simulink model "LQR_bloques_SS_gamma"  (R2023a)
settings: Solver=VariableStepAuto  StartTime=0.0  StopTime=500  RelTol=1e-6
undefined symbols (not defined in the file): A, A_model, A_motor, B, B_mag0, B_model, B_model2, B_motor, C_model, C_model2, C_motor, D_model, D_motor, Gamma, I, J, juliandate, K1, K1_2, K2, K2_2, K3, K_gamma, Ke, Kt, La, n_cal, R_mgt, Ra, T_ext, T_max, T_max_mgt, x0
libraries: slpidlib x12, matrix_library x10, simulink_extras x5, sharedutil x3, aerolibutil x2, vrlib x2, aerolibcubesatveh x1, aerolibgravity2 x1
(part 1 of 2)
settings Model: Creator=Personal  LastModifiedBy=ASUS
settings SolverCC: ZeroCrossAlgorithm=Adaptive
settings DebuggingCC: MaskedZcDiagnostic=none  IgnoredZcDiagnostic=none

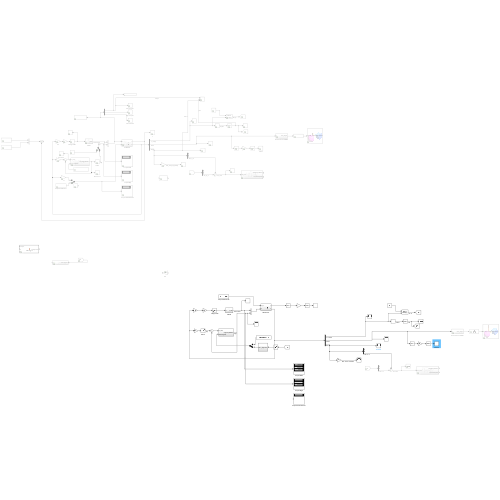
[thumbnail: Simulink's stored preview of the top-level diagram]
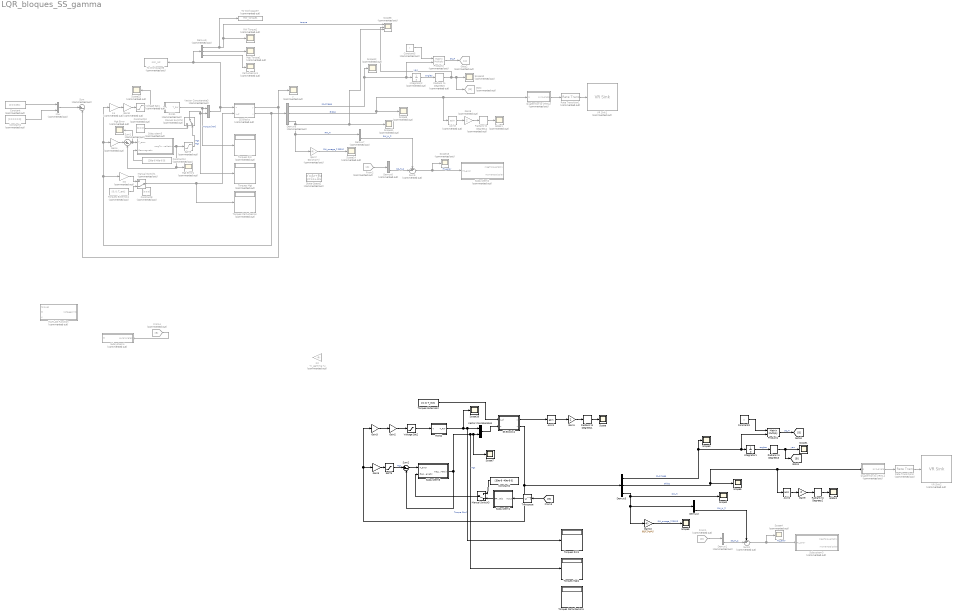
== system LQR_bloques_SS_gamma ==
  Asin1 : Trigonometry  Operator=asin
  Asin2 : Trigonometry  Operator=asin
  Asin3 : Trigonometry  Commented=on  Operator=asin
  Constant : Constant  Commented=on  Value=[0 0 0.05 ]
  Constant1 : Constant  Commented=on  Value=[0 0 0 0 0 0]
  Constant10 : Constant  Commented=on  Value=[0;0;0]
  Constant12 : Constant  Commented=on  Value=[30e-6 40e-6 0]
  Constant2 : Constant  Value=[30e-6 -40e-6 0]
  Constant3 : Constant  Value=I
  Constant5 : Constant  Commented=on  Value=I
  Constant8 : Constant  Commented=on  Value=[0;0;0]
  Demux{1,6..9} (5 alike) : Demux  Commented=on  Outputs=3
  Demux2 : Demux  Outputs=3
  Demux3 : Demux  Outputs=3
  From1 : From  Commented=on  GotoTag=D
  From2 : From  Commented=on
  From4 : From  Commented=on  GotoTag=B
  Gain1 : Gain  Gain=2
  Gain10 : Gain  Gain=60/(2*pi*J)
  Gain2 : Gain  Gain=Ra/Kt
  Gain3 : Gain  Gain=-K1_2  Multiplication=Matrix(K*u)
  Gain4 : Gain  Commented=on  Gain=-K2  Multiplication=Matrix(K*u)
  Gain5 : Gain  Gain=-K2_2  Multiplication=Matrix(K*u)
  Gain6 : Gain  Commented=on  Gain=2
  Gain7 : Gain  Commented=on  Gain=60/(2*pi*J)
  Gain8 : Gain  Commented=on  Gain=Ra/Kt
  Gain9 : Gain  Gain=2
  Gibbs1 : Scope  Commented=on
  Gibbs2 : Scope
  Goto : Goto  Commented=on  GotoTag=B
  Goto2 : Goto  Commented=on
  Integrator1 : Integrator  InitialCondition=[0 0 0]
  Integrator2 : Integrator  Commented=on  InitialCondition=[0 0 0]
  K2 : Gain  Commented=on  Gain=-K_gamma  Multiplication=Matrix(K*u)
  K4 : Gain  Commented=on  Gain=-K1  Multiplication=Matrix(K*u)
  K6 : Gain  Commented=on  Gain=-K3  Multiplication=Matrix(K*u)
  MATLAB Function : MATLAB Function  Commented=on  TreatAsAtomicUnit=on
  Manual Switch1 : ManualSwitch  Commented=on  CurrentSetting=0
  Manual Switch2 : ManualSwitch  Commented=on  CurrentSetting=0
  Manual Switch3 : ManualSwitch  CurrentSetting=0
  Mgt Error : Scope  Commented=on
  Mgt Error1 : Scope  Commented=on
  Mgt Torque1 : Scope  Commented=on
  Mux : Mux  Commented=on  Inputs=2
  Perturbacion1 : Scope  Commented=on
  Product1 : Product  Multiplication=Matrix(*)
  Product2 : Product  Commented=on  Multiplication=Matrix(*)
  Quaternion to VRML1 : Subsystem  Commented=on
  Quaternion to VRML2 : Subsystem  Commented=on
  RW Torque1 : Scope  Commented=on
  RWS1 : Subsystem  Commented=on
  RWS2 : Subsystem
  Radians to Degrees1 : simulink_extras/Transformations/Radians to Degrees
  Radians to Degrees2 : simulink_extras/Transformations/Radians to Degrees
  Radians to Degrees3 : simulink_extras/Transformations/Radians to Degrees
  Radians to Degrees4 : simulink_extras/Transformations/Radians to Degrees  Commented=on
  Radians to Degrees5 : simulink_extras/Transformations/Radians to Degrees  Commented=on
  Rate Transition1 : RateTransition  Commented=on
  Rate Transition2 : RateTransition  Commented=on
  SS Blocks : Subsystem  Commented=on
  SS Blocks1 : Subsystem
  SatT3 : Saturate  Commented=on  UpperLimit=T_max_mgt  LowerLimit=-T_max_mgt
  SatT5 : Saturate  UpperLimit=T_max_mgt  LowerLimit=-T_max_mgt
  Scope{,1..3,5..7,16} (8 alike) : Scope
  Scope{4,9..15} (8 alike) : Scope  Commented=on
  Scope8 : Scope  Commented=on  NumInputPorts=3
  State-Space2 : StateSpace  Commented=on  A=A_model  B=B_model  C=C_model  D=D_model  InitialCondition=x0
  Subsystem1 : Subsystem
  Subsystem2 : Subsystem  Commented=on
  Subsystem3 : Subsystem  Commented=on
  Subsystem4 : Subsystem  Commented=on
  Subsystem5 : Subsystem  Commented=on
  Subsystem6 : Subsystem
  Sum : Sum  Commented=on  Inputs=|+-
  Sum1 : Sum  Commented=on  Inputs=|+-
  Sum2 : Sum  Inputs=|+-
  Sum3 : Sum  Commented=on  Inputs=+-|
  Sum5 : Sum  Commented=on  Inputs=+-|
  To Workspace6 : ToWorkspace  Commented=on  VariableName=sim_U2  SaveFormat=Structure With Time  SampleTime=-1
  To Workspace7 : ToWorkspace  Commented=on  VariableName=RW_torque1  SaveFormat=Structure With Time  SampleTime=-1
  Torques Externos1 : Constant  Commented=on  Value=[0; 0; T_ext]
  Torques Externos2 : Constant  Value=[0; 0; T_ext]
  Torques Mgt : Display  Commented=on
  Torques Mgt1 : Display
  Torques Perturbacion : Display  Commented=on
  Torques Perturbacion1 : Display
  Torques RW : Display  Commented=on
  Torques RW1 : Display
  Transpose : Math  Operator=transpose
  VR Sink1 : vrlib/VR Sink  Commented=on  InstantiateOnLoad=on  SampleTime=0.1  ViewEnable=on  RemoteChange=off  RemoteView=off  FieldsWritten=STLB_Transform.rotation.4.1.1.double  WorldFileName=EscenarioCubeSat.x3d  AutoView=off  VideoDimensions=[]  AllowVariableSize=off  FigureProperties=[]
  VR Sink2 : vrlib/VR Sink  Commented=on  InstantiateOnLoad=on  SampleTime=0.1  ViewEnable=on  RemoteChange=off  RemoteView=off  FieldsWritten=STLB_Transform.rotation.4.1.1.double  WorldFileName=EscenarioCubeSat.x3d  AutoView=off  VideoDimensions=[]  AllowVariableSize=off  FigureProperties=[]
  Vector Concatenate1 : Concatenate
  Vector Concatenate3 : Concatenate  Commented=on
  Voltage Sat1 : Saturate  Commented=on  UpperLimit=6  LowerLimit=-6
  Voltage Sat2 : Saturate  UpperLimit=6  LowerLimit=-6
  y : Scope  Commented=on
  wires:
  Integrator2/1 -> Radians to Degrees5/1  "angles"
  Gain7/1 -> Scope14/1  "RW_omega_Z [RPM]"
  Constant5/1 -> Product2/1
  From4/1 -> Subsystem4/1(euler angles)
  SatT3/1 -> Manual Switch2/2  "Mgt"
  Gain8/1 -> Voltage Sat1/1
  Quaternion to VRML2/1(axis_angle) -> Rate Transition1/1
  From2/1 -> Demux6/1
  Constant10/1 -> Manual Switch2/1
  Asin3/1 -> Gain6/1
  Product2/1 -> Goto2/1  "SC_H"
  Radians to Degrees5/1 -> Scope8/2, Goto/1, Scope10/1  "yaw"
  Demux8/3 -> Scope8/3, Scope11/1, Gain7/1, Demux7/1  "RW_H"
  Demux8/1 -> Integrator2/1, Product2/2, Scope12/1  "sc_omega"
  Voltage Sat1/1 -> Scope15/1, RWS1/1(V)
  Demux7/3 -> Sum5/1  "RW_H_Z"
  Radians to Degrees4/1 -> Gibbs1/1
  Demux9/1 -> To Workspace7/1, Scope8/1, RW Torque1/1  "torque"
  K4/1 -> Gain8/1
  Torques Externos1/1 -> Manual Switch1/2
  Sum5/1 -> Scope13/1, Subsystem2/1(Hz_error)  "Hz_error"
  Demux6/3 -> Sum5/2  "SC_H_Z"
  Rate Transition1/1 -> VR Sink1/1
  Gain6/1 -> Radians to Degrees4/1
  Demux8/2 -> Asin3/1, Quaternion to VRML2/1(q), Scope9/1  "Gibbs"
  RWS1/1(T_RW) -> Torques RW/1, Vector Concatenate3/1  "Torque [Nm]"
  Demux9/2 -> Mgt Torque1/1
  K6/1 -> Manual Switch1/1
  Demux9/3 -> Perturbacion1/1
  Vector Concatenate3/1 -> To Workspace6/1, Demux9/1, SS Blocks/1(u)
  Manual Switch2/1 -> Vector Concatenate3/2, Torques Mgt/1  "Mgt"
  Manual Switch1/1 -> SS Blocks/2(u_d), Torques Perturbacion/1
  SS Blocks/2(x) -> K6/1, K4/1, Gain4/1, Demux8/1
  SS Blocks/1(y) -> Sum/2, y/1
  Constant/1 -> Mux/1
  Constant1/1 -> Mux/2
  Mux/1 -> Sum/1
  Sum1/1 -> Mgt Error/1, Subsystem5/1(T_error)
  Gain4/1 -> Sum1/1
  Subsystem5/1(magTorqueMatrix) -> SatT3/1, Mgt Error1/1, Sum1/2
  Constant12/1 -> Subsystem5/2(Geomagnetic)
  Torques Externos2/1 -> SS Blocks1/1(u_d)
  SS Blocks1/1(y) -> Asin1/1
  Gain1/1 -> Radians to Degrees1/1
  Asin1/1 -> Gain1/1
  Radians to Degrees1/1 -> Scope/1
  SS Blocks1/2(x) -> Demux3/1, Gain3/1, Gain5/1
  Gain5/1 -> SatT5/1
  Gain3/1 -> Gain2/1
  Gain2/1 -> Voltage Sat2/1
  Voltage Sat2/1 -> RWS2/1(V)
  RWS2/1(T_RW) -> Scope16/1, Torques RW1/1, Vector Concatenate1/1  "Torque [Nm]"
  Sum2/1 -> Subsystem6/1(T_error)
  Subsystem6/1(magTorqueMatrix) -> Sum2/2, Torques Mgt1/1, Scope7/1, Vector Concatenate1/2  "Mgt"
  Vector Concatenate1/1 -> SS Blocks1/2(u)
  Demux2/3 -> Sum3/1  "RW_H_Z"
  Demux3/1 -> Integrator1/1, Product1/2, Scope3/1  "sc_omega"
  Demux3/3 -> Scope2/1, Gain10/1, Demux2/1  "RW_H"
  Sum3/1 -> Scope4/1, Subsystem3/1(Hz_error)  "Hz_error"
  Gain9/1 -> Radians to Degrees2/1
  Demux1/3 -> Sum3/2  "SC_H_Z"
  Product1/1 -> [D]  "SC_H"
  Demux3/2 -> Asin2/1, Quaternion to VRML1/1(q), Scope6/1  "Gibbs"
  Radians to Degrees2/1 -> Gibbs2/1
  Rate Transition2/1 -> VR Sink2/1
  Quaternion to VRML1/1(axis_angle) -> Rate Transition2/1
  Constant3/1 -> Product1/1
  Asin2/1 -> Gain9/1
  Radians to Degrees3/1 -> [B], Scope1/1  "yaw"
  From1/1 -> Demux1/1
  Gain10/1 -> Scope5/1  "RW_omega_Z [RPM]"
  Integrator1/1 -> Radians to Degrees3/1  "angles"
  SatT5/1 -> Sum2/1  "Mgt"
  Constant2/1 -> Manual Switch3/1
  Manual Switch3/1 -> Subsystem6/2(Geomagnetic)
  Subsystem1/1(RPY_Magnetic) -> Manual Switch3/2
  Transpose/1 -> Subsystem1/1(Input)
  [B] -> Transpose/1

== system LQR_bloques_SS_gamma/Quaternion to VRML1 ==
  q : Inport
  Asin1 : Trigonometry  Operator=asin
  Constant : Constant  Value=pi/2
  Demux : Demux  Outputs=3
  "Flip 180 deg, rotate 90" : Constant  Value=[0 0.2 0 0]
  Gain2 : Gain  Gain=2
  Mux : Mux
  Quaternion Multiplication : aerolibutil/Quaternion Multiplication
  Saturation : Saturate
  Selector1 : Selector  InputPortWidth=4  IndexOptions=Index vector (dialog)  Indices=[2 3 1 4]  OutputSizes=1
  Sum : Sum  Inputs=|+-
  axis_angle : Outport  VectorParamsAs1DForOutWhenUnconnected=off
  wires:
  Constant/1 -> Sum/1
  Saturation/1 -> Asin1/1
  Asin1/1 -> Gain2/1
  Demux/3 -> Mux/3, Saturation/1
  Gain2/1 -> Mux/4
  Selector1/1 -> axis_angle/1
  Mux/1 -> Selector1/1
  Demux/1 -> Mux/1
  q/1 -> Demux/1
  "Flip 180 deg, rotate 90"/1 -> Quaternion Multiplication/2
  Demux/2 -> Mux/2

== system LQR_bloques_SS_gamma/Quaternion to VRML2 ==
  q : Inport
  Asin1 : Trigonometry  Operator=asin
  Constant : Constant  Value=pi/2
  Demux : Demux  Outputs=3
  "Flip 180 deg, rotate 90" : Constant  Value=[0 0.2 0 0]
  Gain2 : Gain  Gain=2
  Mux : Mux
  Quaternion Multiplication : aerolibutil/Quaternion Multiplication
  Saturation : Saturate
  Selector1 : Selector  InputPortWidth=4  IndexOptions=Index vector (dialog)  Indices=[2 3 1 4]  OutputSizes=1
  Sum : Sum  Inputs=|+-
  axis_angle : Outport  VectorParamsAs1DForOutWhenUnconnected=off
  wires:
  Constant/1 -> Sum/1
  Saturation/1 -> Asin1/1
  Asin1/1 -> Gain2/1
  Demux/3 -> Mux/3, Saturation/1
  Gain2/1 -> Mux/4
  Selector1/1 -> axis_angle/1
  Mux/1 -> Selector1/1
  Demux/1 -> Mux/1
  q/1 -> Demux/1
  "Flip 180 deg, rotate 90"/1 -> Quaternion Multiplication/2
  Demux/2 -> Mux/2

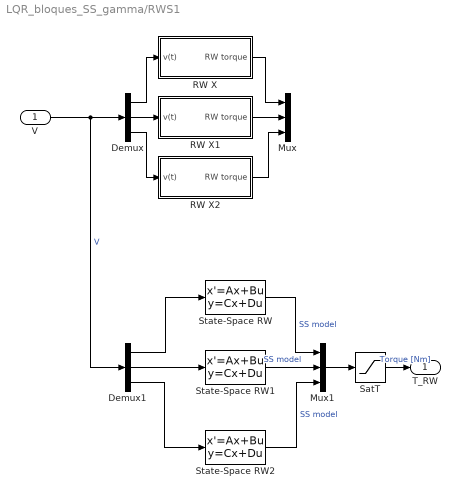
== system LQR_bloques_SS_gamma/RWS1 ==
  V : Inport
  Demux : Demux  Outputs=3
  Demux1 : Demux  Outputs=3
  Mux : Mux  Inputs=3
  Mux1 : Mux  Inputs=3
  RW X : Subsystem
  RW X1 : Subsystem
  RW X2 : Subsystem
  SatT : Saturate  UpperLimit=T_max  LowerLimit=-T_max
  State-Space RW : StateSpace  A=A_motor  B=B_motor  C=C_motor  D=D_motor  InitialCondition=0
  State-Space RW1 : StateSpace  A=A_motor  B=B_motor  C=C_motor  D=D_motor  InitialCondition=0
  State-Space RW2 : StateSpace  A=A_motor  B=B_motor  C=C_motor  D=D_motor  InitialCondition=0
  T_RW : Outport
  wires:
  Demux/1 -> RW X/1(v(t))
  V/1 -> Demux1/1, Demux/1  "V"
  Demux/3 -> RW X2/1(v(t))
  Demux/2 -> RW X1/1(v(t))
  RW X1/1(RW torque) -> Mux/2
  RW X2/1(RW torque) -> Mux/3
  RW X/1(RW torque) -> Mux/1
  Demux1/1 -> State-Space RW/1
  Demux1/2 -> State-Space RW1/1
  Demux1/3 -> State-Space RW2/1
  State-Space RW1/1 -> Mux1/2  "SS model"
  State-Space RW/1 -> Mux1/1  "SS model"
  State-Space RW2/1 -> Mux1/3  "SS model"
  Mux1/1 -> SatT/1
  SatT/1 -> T_RW/1  "Torque [Nm]"

== system LQR_bloques_SS_gamma/RWS2 ==
  V : Inport
  Demux : Demux  Outputs=3
  Demux1 : Demux  Outputs=3
  Mux : Mux  Inputs=3
  Mux1 : Mux  Inputs=3
  RW X : Subsystem
  RW X1 : Subsystem
  RW X2 : Subsystem
  SatT : Saturate  UpperLimit=T_max  LowerLimit=-T_max
  State-Space RW : StateSpace  A=A_motor  B=B_motor  C=C_motor  D=D_motor  InitialCondition=0
  State-Space RW1 : StateSpace  A=A_motor  B=B_motor  C=C_motor  D=D_motor  InitialCondition=0
  State-Space RW2 : StateSpace  A=A_motor  B=B_motor  C=C_motor  D=D_motor  InitialCondition=0
  T_RW : Outport
  wires:
  Demux/1 -> RW X/1(v(t))
  V/1 -> Demux1/1, Demux/1  "V"
  Demux/3 -> RW X2/1(v(t))
  Demux/2 -> RW X1/1(v(t))
  RW X1/1(RW torque) -> Mux/2
  RW X2/1(RW torque) -> Mux/3
  RW X/1(RW torque) -> Mux/1
  Demux1/1 -> State-Space RW/1
  Demux1/2 -> State-Space RW1/1
  Demux1/3 -> State-Space RW2/1
  State-Space RW1/1 -> Mux1/2  "SS model"
  State-Space RW/1 -> Mux1/1  "SS model"
  State-Space RW2/1 -> Mux1/3  "SS model"
  Mux1/1 -> SatT/1
  SatT/1 -> T_RW/1  "Torque [Nm]"

== system LQR_bloques_SS_gamma/SS Blocks ==
  u : Inport
  u_d : Inport  Port=2
  A : Gain  Gain=A_model  Multiplication=Matrix(K*u)
  B : Gain  Gain=B_model2  Multiplication=Matrix(K*u)
  B1 : Gain  Gain=Gamma  Multiplication=Matrix(K*u)
  C : Gain  Gain=C_model2  Multiplication=Matrix(K*u)
  Integrator : Integrator  InitialCondition=x0
  Sum : Sum  Inputs=+++
  y : Outport
  x : Outport  Port=2
  wires:
  B/1 -> Sum/2
  u/1 -> B/1
  Sum/1 -> Integrator/1  "x_dot"
  A/1 -> Sum/3
  C/1 -> y/1
  Integrator/1 -> C/1, x/1, A/1
  u_d/1 -> B1/1
  B1/1 -> Sum/1

== system LQR_bloques_SS_gamma/SS Blocks1 ==
  u_d : Inport
  u : Inport  Port=2
  A : Gain  Gain=A_model  Multiplication=Matrix(K*u)
  B : Gain  Gain=B_model2  Multiplication=Matrix(K*u)
  C : Gain  Gain=C_model2  Multiplication=Matrix(K*u)
  Gamma : Gain  Gain=Gamma  Multiplication=Matrix(K*u)
  Integrator : Integrator  InitialCondition=x0
  Sum : Sum  Inputs=+++
  y : Outport
  x : Outport  Port=2
  wires:
  B/1 -> Sum/2
  u/1 -> B/1
  Sum/1 -> Integrator/1  "x_dot"
  A/1 -> Sum/3
  C/1 -> y/1
  Integrator/1 -> C/1, x/1, A/1
  u_d/1 -> Gamma/1
  Gamma/1 -> Sum/1

== system LQR_bloques_SS_gamma/Subsystem1 ==
  Input : Inport
  Clock : Clock
  Constant1 : Constant  Value=B_mag0
  Extract B : MATLAB Function  TreatAsAtomicUnit=on
  MATLAB Function : MATLAB Function  TreatAsAtomicUnit=on
  Scope8 : Scope
  Zero-Order Hold : ZeroOrderHold  SampleTime=-1
  RPY_Magnetic : Outport
  wires:
  Constant1/1 -> Extract B/1(B_cal)
  Extract B/1(XYZ_Magnetic) -> MATLAB Function/1(NEDMagnetic), Scope8/1
  Input/1 -> MATLAB Function/2(RPY)
  Zero-Order Hold/1 -> Extract B/2(time)
  MATLAB Function/1(RPY_Magnetic) -> RPY_Magnetic/1
  Clock/1 -> Zero-Order Hold/1

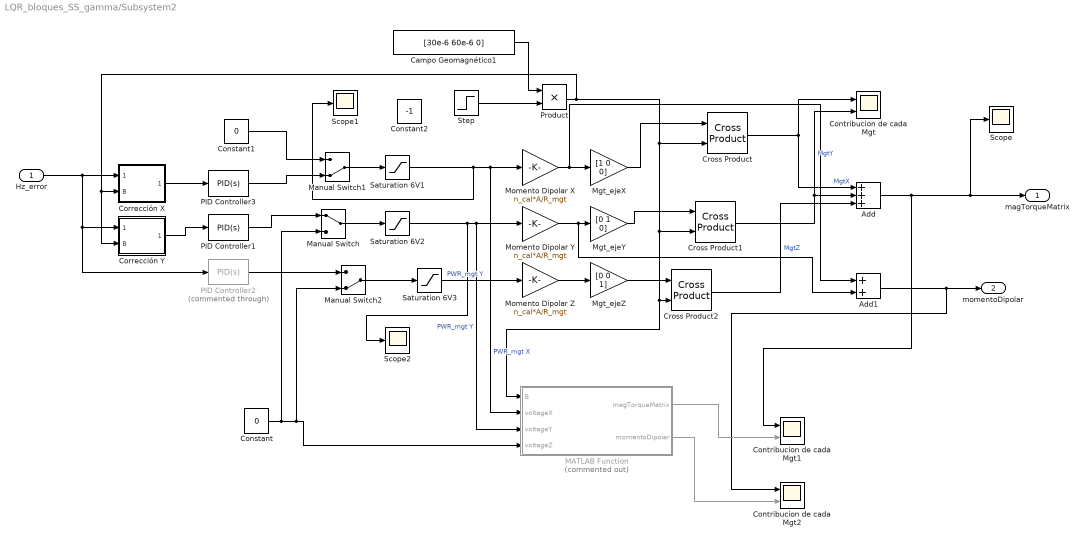
== system LQR_bloques_SS_gamma/Subsystem2 ==
  Hz_error : Inport
  Add : Sum  Inputs=+++
  Add1 : Sum
  Campo Geomagnético1 : Constant  Value=[30e-6 60e-6 0]
  Constant : Constant  Value=0
  Constant1 : Constant  Value=0
  Constant2 : Constant  Value=-1
  Contribucion de cada Mgt : Scope  NumInputPorts=2
  Contribucion de cada Mgt1 : Scope  NumInputPorts=2
  Contribucion de cada Mgt2 : Scope  NumInputPorts=2
  Corrección X : MATLAB Function  TreatAsAtomicUnit=on
  Corrección Y : MATLAB Function  TreatAsAtomicUnit=on
  Cross Product : matrix_library/Cross Product
  Cross Product1 : matrix_library/Cross Product
  Cross Product2 : matrix_library/Cross Product
  MATLAB Function : MATLAB Function  Commented=on  TreatAsAtomicUnit=on
  Manual Switch : ManualSwitch
  Manual Switch1 : ManualSwitch  CurrentSetting=0
  Manual Switch2 : ManualSwitch  CurrentSetting=0
  Mgt_ejeX : Gain  Gain=[1 0 0]
  Mgt_ejeY : Gain  Gain=[0 1 0]
  Mgt_ejeZ : Gain  Gain=[0 0 1]
  Momento Dipolar X : Gain  Gain=n_cal*A/R_mgt
  Momento Dipolar Y : Gain  Gain=n_cal*A/R_mgt
  Momento Dipolar Z : Gain  Gain=n_cal*A/R_mgt
  PID Controller1 : slpidlib/PID Controller  Controller=PID  Form=Parallel  TimeDomain=Continuous-time  UseExternalTs=off  SampleTime=-1  IntegratorMethod=Forward Euler  FilterMethod=Forward Euler  ControllerParametersSource=internal  P=4500  I=800  UseKiTs=off  D=8000  N=100  UseFilter=on  TunerSelectOption=Transfer Function Based (PID Tuner App)  InitialConditionSource=internal  InitialConditionForIntegrator=0  InitialConditionForFilter=0  DifferentiatorICPrevScaledInput=0  ExternalReset=none  TrackingMode=off  Kt=1  LimitOutput=off  SatLimitsSource=internal  UpperSaturationLimit=1  LowerSaturationLimit=-1  LinearizeAsGain=on  AntiWindupMode=none  Kb=1  LimitIntegrator=off  UpperIntegratorSaturationLimit=inf  LowerIntegratorSaturationLimit=-inf  POutMin=[]  POutMax=[]  IOutMin=[]  IOutMax=[]  DOutMin=[]  DOutMax=[]  NOutMin=[]  NOutMax=[]  SumOutMin=[]  SumOutMax=[]  SaturationOutMin=[]  SaturationOutMax=[]  PParamMin=[]  PParamMax=[]  IParamMin=[]  IParamMax=[]  DParamMin=[]  DParamMax=[]  NParamMin=[]  NParamMax=[]  KbParamMin=[]  KbParamMax=[]  KtParamMin=[]  KtParamMax=[]  KbOutMin=[]  KbOutMax=[]  KtOutMin=[]  KtOutMax=[]  IntegratorOutMin=[]  IntegratorOutMax=[]  FilterOutMin=[]  FilterOutMax=[]  SumI1OutMin=[]  SumI1OutMax=[]  SumI2OutMin=[]  SumI2OutMax=[]  SumI3OutMin=[]  SumI3OutMax=[]  SumI4OutMin=[]  SumI4OutMax=[]  SumDOutMin=[]  SumDOutMax=[]  DifferentiatorOutMin=[]  DifferentiatorOutMax=[]  FilterDiffOutCoefMin=[]  FilterDiffOutCoefMax=[]  ReciprocalOutMin=[]  ReciprocalOutMax=[]  SumDenOutMin=[]  SumDenOutMax=[]  SumNumOutMin=[]  SumNumOutMax=[]  DivideOutMin=[]  DivideOutMax=[]  UdiffTsProdOutMin=[]  UdiffTsProdOutMax=[]  NTsProdOutMin=[]  NTsProdOutMax=[]  UintegralTsProdOutMin=[]  UintegralTsProdOutMax=[]  UngainTsProdOutMin=[]  UngainTsProdOutMax=[]  ClampingZeroOutDataTypeStr=Inherit: Inherit via back propagation  ClampingZeroOutMin=[]  ClampingZeroOutMax=[]  FilterDenConstantOutDataTypeStr=Inherit: Inherit via back propagation  FilterDenConstantOutMin=[]  FilterDenConstantOutMax=[]  PCopyOutDataTypeStr=Inherit: Inherit via back propagation  PCopyOutMin=[]  PCopyOutMax=[]  NCopyOutDataTypeStr=Inherit: Inherit via back propagation  NCopyOutMin=[]  NCopyOutMax=[]  IntegratorContinuousStateAttributes=''  IntegratorStateMustResolveToSignalObject=off  IntegratorRTWStateStorageClass=Auto  FilterContinuousStateAttributes=''  FilterStateMustResolveToSignalObject=off  FilterRTWStateStorageClass=Auto  ParallelPVariant=InternalParameters  IdealPVariant=Disabled  IVariant=InternalParameters  DVariant=InternalParameters  IntegratorVariant=Continuous  SatVariant=Disabled  AWVariant=Passthrough  PCopyVariant=Disabled  TRVariant=Disabled  FdbkBlocksVariant=Forward  IdealPFdbkVariant=Disabled  SatFdbkVariant=Disabled  DerivativeFilterVariant=ContFilter  NVariant=InternalParameters  NCopyVariant=Disabled  FilterICVariant=InternalICsFilter  IntegratorICVariant=InternalICs  ExternalResetVariant=Disabled  TRSumVariant=Passthrough  SumFdbkVariant=Disabled  SumVariant=Sum_PID  TsampFilterVariant=InternalTs  TsampNgainVariant=Passthrough  TsampIntegralVariant=Disabled_SignalSpec  ExternalSaturationOutDataTypeStr=Inherit: Same as second input
  PID Controller2 : slpidlib/PID Controller  Commented=through  Controller=PID  Form=Parallel  TimeDomain=Continuous-time  UseExternalTs=off  SampleTime=-1  IntegratorMethod=Forward Euler  FilterMethod=Forward Euler  ControllerParametersSource=internal  P=4500  I=800  UseKiTs=off  D=8000  N=100  UseFilter=on  TunerSelectOption=Transfer Function Based (PID Tuner App)  InitialConditionSource=internal  InitialConditionForIntegrator=0  InitialConditionForFilter=0  DifferentiatorICPrevScaledInput=0  ExternalReset=none  TrackingMode=off  Kt=1  LimitOutput=off  SatLimitsSource=internal  UpperSaturationLimit=1  LowerSaturationLimit=-1  LinearizeAsGain=on  AntiWindupMode=none  Kb=1  LimitIntegrator=off  UpperIntegratorSaturationLimit=inf  LowerIntegratorSaturationLimit=-inf  POutMin=[]  POutMax=[]  IOutMin=[]  IOutMax=[]  DOutMin=[]  DOutMax=[]  NOutMin=[]  NOutMax=[]  SumOutMin=[]  SumOutMax=[]  SaturationOutMin=[]  SaturationOutMax=[]  PParamMin=[]  PParamMax=[]  IParamMin=[]  IParamMax=[]  DParamMin=[]  DParamMax=[]  NParamMin=[]  NParamMax=[]  KbParamMin=[]  KbParamMax=[]  KtParamMin=[]  KtParamMax=[]  KbOutMin=[]  KbOutMax=[]  KtOutMin=[]  KtOutMax=[]  IntegratorOutMin=[]  IntegratorOutMax=[]  FilterOutMin=[]  FilterOutMax=[]  SumI1OutMin=[]  SumI1OutMax=[]  SumI2OutMin=[]  SumI2OutMax=[]  SumI3OutMin=[]  SumI3OutMax=[]  SumI4OutMin=[]  SumI4OutMax=[]  SumDOutMin=[]  SumDOutMax=[]  DifferentiatorOutMin=[]  DifferentiatorOutMax=[]  FilterDiffOutCoefMin=[]  FilterDiffOutCoefMax=[]  ReciprocalOutMin=[]  ReciprocalOutMax=[]  SumDenOutMin=[]  SumDenOutMax=[]  SumNumOutMin=[]  SumNumOutMax=[]  DivideOutMin=[]  DivideOutMax=[]  UdiffTsProdOutMin=[]  UdiffTsProdOutMax=[]  NTsProdOutMin=[]  NTsProdOutMax=[]  UintegralTsProdOutMin=[]  UintegralTsProdOutMax=[]  UngainTsProdOutMin=[]  UngainTsProdOutMax=[]  ClampingZeroOutDataTypeStr=Inherit: Inherit via back propagation  ClampingZeroOutMin=[]  ClampingZeroOutMax=[]  FilterDenConstantOutDataTypeStr=Inherit: Inherit via back propagation  FilterDenConstantOutMin=[]  FilterDenConstantOutMax=[]  PCopyOutDataTypeStr=Inherit: Inherit via back propagation  PCopyOutMin=[]  PCopyOutMax=[]  NCopyOutDataTypeStr=Inherit: Inherit via back propagation  NCopyOutMin=[]  NCopyOutMax=[]  IntegratorContinuousStateAttributes=''  IntegratorStateMustResolveToSignalObject=off  IntegratorRTWStateStorageClass=Auto  FilterContinuousStateAttributes=''  FilterStateMustResolveToSignalObject=off  FilterRTWStateStorageClass=Auto  ParallelPVariant=InternalParameters  IdealPVariant=Disabled  IVariant=InternalParameters  DVariant=InternalParameters  IntegratorVariant=Continuous  SatVariant=Disabled  AWVariant=Passthrough  PCopyVariant=Disabled  TRVariant=Disabled  FdbkBlocksVariant=Forward  IdealPFdbkVariant=Disabled  SatFdbkVariant=Disabled  DerivativeFilterVariant=ContFilter  NVariant=InternalParameters  NCopyVariant=Disabled  FilterICVariant=InternalICsFilter  IntegratorICVariant=InternalICs  ExternalResetVariant=Disabled  TRSumVariant=Passthrough  SumFdbkVariant=Disabled  SumVariant=Sum_PID  TsampFilterVariant=InternalTs  TsampNgainVariant=Passthrough  TsampIntegralVariant=Disabled_SignalSpec  ExternalSaturationOutDataTypeStr=Inherit: Same as second input
  PID Controller3 : slpidlib/PID Controller  Controller=PID  Form=Parallel  TimeDomain=Continuous-time  UseExternalTs=off  SampleTime=-1  IntegratorMethod=Forward Euler  FilterMethod=Forward Euler  ControllerParametersSource=internal  P=4500  I=800  UseKiTs=off  D=8000  N=100  UseFilter=on  TunerSelectOption=Transfer Function Based (PID Tuner App)  InitialConditionSource=internal  InitialConditionForIntegrator=0  InitialConditionForFilter=0  DifferentiatorICPrevScaledInput=0  ExternalReset=none  TrackingMode=off  Kt=1  LimitOutput=off  SatLimitsSource=internal  UpperSaturationLimit=1  LowerSaturationLimit=-1  LinearizeAsGain=on  AntiWindupMode=none  Kb=1  LimitIntegrator=off  UpperIntegratorSaturationLimit=inf  LowerIntegratorSaturationLimit=-inf  POutMin=[]  POutMax=[]  IOutMin=[]  IOutMax=[]  DOutMin=[]  DOutMax=[]  NOutMin=[]  NOutMax=[]  SumOutMin=[]  SumOutMax=[]  SaturationOutMin=[]  SaturationOutMax=[]  PParamMin=[]  PParamMax=[]  IParamMin=[]  IParamMax=[]  DParamMin=[]  DParamMax=[]  NParamMin=[]  NParamMax=[]  KbParamMin=[]  KbParamMax=[]  KtParamMin=[]  KtParamMax=[]  KbOutMin=[]  KbOutMax=[]  KtOutMin=[]  KtOutMax=[]  IntegratorOutMin=[]  IntegratorOutMax=[]  FilterOutMin=[]  FilterOutMax=[]  SumI1OutMin=[]  SumI1OutMax=[]  SumI2OutMin=[]  SumI2OutMax=[]  SumI3OutMin=[]  SumI3OutMax=[]  SumI4OutMin=[]  SumI4OutMax=[]  SumDOutMin=[]  SumDOutMax=[]  DifferentiatorOutMin=[]  DifferentiatorOutMax=[]  FilterDiffOutCoefMin=[]  FilterDiffOutCoefMax=[]  ReciprocalOutMin=[]  ReciprocalOutMax=[]  SumDenOutMin=[]  SumDenOutMax=[]  SumNumOutMin=[]  SumNumOutMax=[]  DivideOutMin=[]  DivideOutMax=[]  UdiffTsProdOutMin=[]  UdiffTsProdOutMax=[]  NTsProdOutMin=[]  NTsProdOutMax=[]  UintegralTsProdOutMin=[]  UintegralTsProdOutMax=[]  UngainTsProdOutMin=[]  UngainTsProdOutMax=[]  ClampingZeroOutDataTypeStr=Inherit: Inherit via back propagation  ClampingZeroOutMin=[]  ClampingZeroOutMax=[]  FilterDenConstantOutDataTypeStr=Inherit: Inherit via back propagation  FilterDenConstantOutMin=[]  FilterDenConstantOutMax=[]  PCopyOutDataTypeStr=Inherit: Inherit via back propagation  PCopyOutMin=[]  PCopyOutMax=[]  NCopyOutDataTypeStr=Inherit: Inherit via back propagation  NCopyOutMin=[]  NCopyOutMax=[]  IntegratorContinuousStateAttributes=''  IntegratorStateMustResolveToSignalObject=off  IntegratorRTWStateStorageClass=Auto  FilterContinuousStateAttributes=''  FilterStateMustResolveToSignalObject=off  FilterRTWStateStorageClass=Auto  ParallelPVariant=InternalParameters  IdealPVariant=Disabled  IVariant=InternalParameters  DVariant=InternalParameters  IntegratorVariant=Continuous  SatVariant=Disabled  AWVariant=Passthrough  PCopyVariant=Disabled  TRVariant=Disabled  FdbkBlocksVariant=Forward  IdealPFdbkVariant=Disabled  SatFdbkVariant=Disabled  DerivativeFilterVariant=ContFilter  NVariant=InternalParameters  NCopyVariant=Disabled  FilterICVariant=InternalICsFilter  IntegratorICVariant=InternalICs  ExternalResetVariant=Disabled  TRSumVariant=Passthrough  SumFdbkVariant=Disabled  SumVariant=Sum_PID  TsampFilterVariant=InternalTs  TsampNgainVariant=Passthrough  TsampIntegralVariant=Disabled_SignalSpec  ExternalSaturationOutDataTypeStr=Inherit: Same as second input
  Product : Product
  Saturation 6V1 : Saturate  UpperLimit=5  LowerLimit=-5
  Saturation 6V2 : Saturate  UpperLimit=5  LowerLimit=-5
  Saturation 6V3 : Saturate  UpperLimit=5  LowerLimit=-5
  Scope : Scope
  Scope1 : Scope
  Scope2 : Scope
  Step : Step  Time=0  After=-1  SampleTime=0
  magTorqueMatrix : Outport
  momentoDipolar : Outport  Port=2
  wires:
  Corrección Y/1(H_error) -> PID Controller1/1
  Corrección X/1(H_error) -> PID Controller3/1
  Step/1 -> Product/2
  Campo Geomagnético1/1 -> Product/1
  Cross Product2/1 -> Add/3  "MgtZ"
  Mgt_ejeZ/1 -> Cross Product2/1
  Momento Dipolar Z/1 -> Mgt_ejeZ/1
  Saturation 6V3/1 -> Momento Dipolar Z/1  "PWR_mgt Y"
  PID Controller2/1 -> Manual Switch2/1
  Manual Switch2/1 -> Saturation 6V3/1
  MATLAB Function/2(momentoDipolar) -> Contribucion de cada Mgt2/2
  Add1/1 -> momentoDipolar/1, Contribucion de cada Mgt2/1
  MATLAB Function/1(magTorqueMatrix) -> Contribucion de cada Mgt1/2
  Add/1 -> magTorqueMatrix/1, Scope/1, Contribucion de cada Mgt1/1
  Cross Product1/1 -> Add/2, Contribucion de cada Mgt/2  "MgtY"
  Mgt_ejeY/1 -> Cross Product1/1
  Momento Dipolar Y/1 -> Mgt_ejeY/1, Add1/2
  Saturation 6V2/1 -> Momento Dipolar Y/1, MATLAB Function/3(voltageY), Scope2/1  "PWR_mgt Y"
  Cross Product/1 -> Contribucion de cada Mgt/1, Add/1  "MgtX"
  Mgt_ejeX/1 -> Cross Product/1
  Momento Dipolar X/1 -> Mgt_ejeX/1, Add1/1
  Manual Switch1/1 -> Saturation 6V1/1
  Constant1/1 -> Manual Switch1/1
  Constant/1 -> Manual Switch/2, MATLAB Function/4(voltageZ), Manual Switch2/2
  PID Controller1/1 -> Manual Switch/1
  Manual Switch/1 -> Saturation 6V2/1
  Product/1 -> Cross Product/2, Cross Product1/2, Cross Product2/2, MATLAB Function/1(B), Corrección X/2(B), Corrección Y/2(B)
  Hz_error/1 -> Corrección X/1("H_error "), Corrección Y/1("H_error "), PID Controller2/1
  Saturation 6V1/1 -> Momento Dipolar X/1, MATLAB Function/2(voltageX), Scope1/1  "PWR_mgt X"
  PID Controller3/1 -> Manual Switch1/2

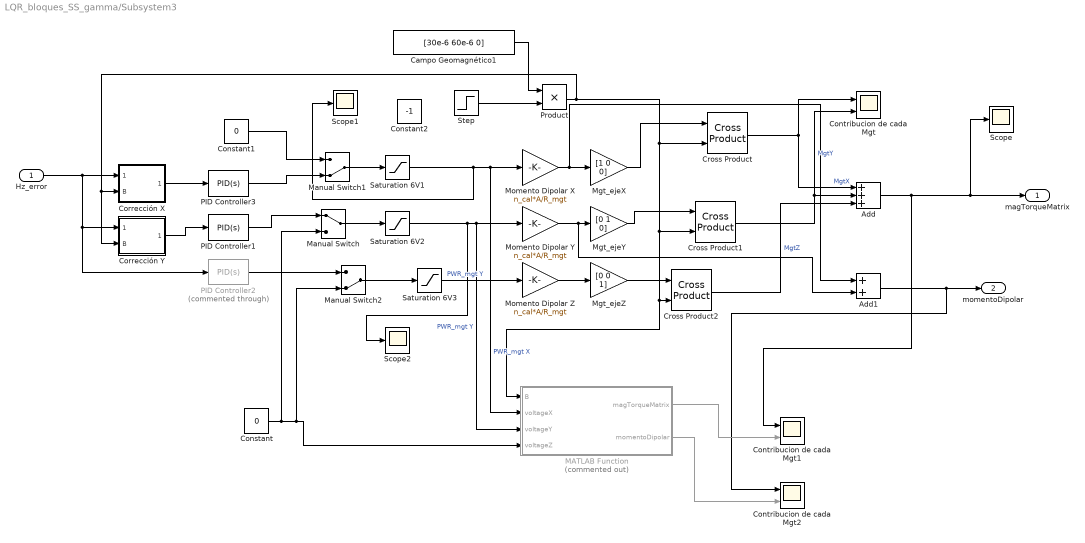
== system LQR_bloques_SS_gamma/Subsystem3 ==
  Hz_error : Inport
  Add : Sum  Inputs=+++
  Add1 : Sum
  Campo Geomagnético1 : Constant  Value=[30e-6 60e-6 0]
  Constant : Constant  Value=0
  Constant1 : Constant  Value=0
  Constant2 : Constant  Value=-1
  Contribucion de cada Mgt : Scope  NumInputPorts=2
  Contribucion de cada Mgt1 : Scope  NumInputPorts=2
  Contribucion de cada Mgt2 : Scope  NumInputPorts=2
  Corrección X : MATLAB Function  TreatAsAtomicUnit=on
  Corrección Y : MATLAB Function  TreatAsAtomicUnit=on
  Cross Product : matrix_library/Cross Product
  Cross Product1 : matrix_library/Cross Product
  Cross Product2 : matrix_library/Cross Product
  MATLAB Function : MATLAB Function  Commented=on  TreatAsAtomicUnit=on
  Manual Switch : ManualSwitch
  Manual Switch1 : ManualSwitch  CurrentSetting=0
  Manual Switch2 : ManualSwitch  CurrentSetting=0
  Mgt_ejeX : Gain  Gain=[1 0 0]
  Mgt_ejeY : Gain  Gain=[0 1 0]
  Mgt_ejeZ : Gain  Gain=[0 0 1]
  Momento Dipolar X : Gain  Gain=n_cal*A/R_mgt
  Momento Dipolar Y : Gain  Gain=n_cal*A/R_mgt
  Momento Dipolar Z : Gain  Gain=n_cal*A/R_mgt
  PID Controller1 : slpidlib/PID Controller  Controller=PID  Form=Parallel  TimeDomain=Continuous-time  UseExternalTs=off  SampleTime=-1  IntegratorMethod=Forward Euler  FilterMethod=Forward Euler  ControllerParametersSource=internal  P=4500  I=800  UseKiTs=off  D=8000  N=100  UseFilter=on  TunerSelectOption=Transfer Function Based (PID Tuner App)  InitialConditionSource=internal  InitialConditionForIntegrator=0  InitialConditionForFilter=0  DifferentiatorICPrevScaledInput=0  ExternalReset=none  TrackingMode=off  Kt=1  LimitOutput=off  SatLimitsSource=internal  UpperSaturationLimit=1  LowerSaturationLimit=-1  LinearizeAsGain=on  AntiWindupMode=none  Kb=1  LimitIntegrator=off  UpperIntegratorSaturationLimit=inf  LowerIntegratorSaturationLimit=-inf  POutMin=[]  POutMax=[]  IOutMin=[]  IOutMax=[]  DOutMin=[]  DOutMax=[]  NOutMin=[]  NOutMax=[]  SumOutMin=[]  SumOutMax=[]  SaturationOutMin=[]  SaturationOutMax=[]  PParamMin=[]  PParamMax=[]  IParamMin=[]  IParamMax=[]  DParamMin=[]  DParamMax=[]  NParamMin=[]  NParamMax=[]  KbParamMin=[]  KbParamMax=[]  KtParamMin=[]  KtParamMax=[]  KbOutMin=[]  KbOutMax=[]  KtOutMin=[]  KtOutMax=[]  IntegratorOutMin=[]  IntegratorOutMax=[]  FilterOutMin=[]  FilterOutMax=[]  SumI1OutMin=[]  SumI1OutMax=[]  SumI2OutMin=[]  SumI2OutMax=[]  SumI3OutMin=[]  SumI3OutMax=[]  SumI4OutMin=[]  SumI4OutMax=[]  SumDOutMin=[]  SumDOutMax=[]  DifferentiatorOutMin=[]  DifferentiatorOutMax=[]  FilterDiffOutCoefMin=[]  FilterDiffOutCoefMax=[]  ReciprocalOutMin=[]  ReciprocalOutMax=[]  SumDenOutMin=[]  SumDenOutMax=[]  SumNumOutMin=[]  SumNumOutMax=[]  DivideOutMin=[]  DivideOutMax=[]  UdiffTsProdOutMin=[]  UdiffTsProdOutMax=[]  NTsProdOutMin=[]  NTsProdOutMax=[]  UintegralTsProdOutMin=[]  UintegralTsProdOutMax=[]  UngainTsProdOutMin=[]  UngainTsProdOutMax=[]  ClampingZeroOutDataTypeStr=Inherit: Inherit via back propagation  ClampingZeroOutMin=[]  ClampingZeroOutMax=[]  FilterDenConstantOutDataTypeStr=Inherit: Inherit via back propagation  FilterDenConstantOutMin=[]  FilterDenConstantOutMax=[]  PCopyOutDataTypeStr=Inherit: Inherit via back propagation  PCopyOutMin=[]  PCopyOutMax=[]  NCopyOutDataTypeStr=Inherit: Inherit via back propagation  NCopyOutMin=[]  NCopyOutMax=[]  IntegratorContinuousStateAttributes=''  IntegratorStateMustResolveToSignalObject=off  IntegratorRTWStateStorageClass=Auto  FilterContinuousStateAttributes=''  FilterStateMustResolveToSignalObject=off  FilterRTWStateStorageClass=Auto  ParallelPVariant=InternalParameters  IdealPVariant=Disabled  IVariant=InternalParameters  DVariant=InternalParameters  IntegratorVariant=Continuous  SatVariant=Disabled  AWVariant=Passthrough  PCopyVariant=Disabled  TRVariant=Disabled  FdbkBlocksVariant=Forward  IdealPFdbkVariant=Disabled  SatFdbkVariant=Disabled  DerivativeFilterVariant=ContFilter  NVariant=InternalParameters  NCopyVariant=Disabled  FilterICVariant=InternalICsFilter  IntegratorICVariant=InternalICs  ExternalResetVariant=Disabled  TRSumVariant=Passthrough  SumFdbkVariant=Disabled  SumVariant=Sum_PID  TsampFilterVariant=InternalTs  TsampNgainVariant=Passthrough  TsampIntegralVariant=Disabled_SignalSpec  ExternalSaturationOutDataTypeStr=Inherit: Same as second input
  PID Controller2 : slpidlib/PID Controller  Commented=through  Controller=PID  Form=Parallel  TimeDomain=Continuous-time  UseExternalTs=off  SampleTime=-1  IntegratorMethod=Forward Euler  FilterMethod=Forward Euler  ControllerParametersSource=internal  P=4500  I=800  UseKiTs=off  D=8000  N=100  UseFilter=on  TunerSelectOption=Transfer Function Based (PID Tuner App)  InitialConditionSource=internal  InitialConditionForIntegrator=0  InitialConditionForFilter=0  DifferentiatorICPrevScaledInput=0  ExternalReset=none  TrackingMode=off  Kt=1  LimitOutput=off  SatLimitsSource=internal  UpperSaturationLimit=1  LowerSaturationLimit=-1  LinearizeAsGain=on  AntiWindupMode=none  Kb=1  LimitIntegrator=off  UpperIntegratorSaturationLimit=inf  LowerIntegratorSaturationLimit=-inf  POutMin=[]  POutMax=[]  IOutMin=[]  IOutMax=[]  DOutMin=[]  DOutMax=[]  NOutMin=[]  NOutMax=[]  SumOutMin=[]  SumOutMax=[]  SaturationOutMin=[]  SaturationOutMax=[]  PParamMin=[]  PParamMax=[]  IParamMin=[]  IParamMax=[]  DParamMin=[]  DParamMax=[]  NParamMin=[]  NParamMax=[]  KbParamMin=[]  KbParamMax=[]  KtParamMin=[]  KtParamMax=[]  KbOutMin=[]  KbOutMax=[]  KtOutMin=[]  KtOutMax=[]  IntegratorOutMin=[]  IntegratorOutMax=[]  FilterOutMin=[]  FilterOutMax=[]  SumI1OutMin=[]  SumI1OutMax=[]  SumI2OutMin=[]  SumI2OutMax=[]  SumI3OutMin=[]  SumI3OutMax=[]  SumI4OutMin=[]  SumI4OutMax=[]  SumDOutMin=[]  SumDOutMax=[]  DifferentiatorOutMin=[]  DifferentiatorOutMax=[]  FilterDiffOutCoefMin=[]  FilterDiffOutCoefMax=[]  ReciprocalOutMin=[]  ReciprocalOutMax=[]  SumDenOutMin=[]  SumDenOutMax=[]  SumNumOutMin=[]  SumNumOutMax=[]  DivideOutMin=[]  DivideOutMax=[]  UdiffTsProdOutMin=[]  UdiffTsProdOutMax=[]  NTsProdOutMin=[]  NTsProdOutMax=[]  UintegralTsProdOutMin=[]  UintegralTsProdOutMax=[]  UngainTsProdOutMin=[]  UngainTsProdOutMax=[]  ClampingZeroOutDataTypeStr=Inherit: Inherit via back propagation  ClampingZeroOutMin=[]  ClampingZeroOutMax=[]  FilterDenConstantOutDataTypeStr=Inherit: Inherit via back propagation  FilterDenConstantOutMin=[]  FilterDenConstantOutMax=[]  PCopyOutDataTypeStr=Inherit: Inherit via back propagation  PCopyOutMin=[]  PCopyOutMax=[]  NCopyOutDataTypeStr=Inherit: Inherit via back propagation  NCopyOutMin=[]  NCopyOutMax=[]  IntegratorContinuousStateAttributes=''  IntegratorStateMustResolveToSignalObject=off  IntegratorRTWStateStorageClass=Auto  FilterContinuousStateAttributes=''  FilterStateMustResolveToSignalObject=off  FilterRTWStateStorageClass=Auto  ParallelPVariant=InternalParameters  IdealPVariant=Disabled  IVariant=InternalParameters  DVariant=InternalParameters  IntegratorVariant=Continuous  SatVariant=Disabled  AWVariant=Passthrough  PCopyVariant=Disabled  TRVariant=Disabled  FdbkBlocksVariant=Forward  IdealPFdbkVariant=Disabled  SatFdbkVariant=Disabled  DerivativeFilterVariant=ContFilter  NVariant=InternalParameters  NCopyVariant=Disabled  FilterICVariant=InternalICsFilter  IntegratorICVariant=InternalICs  ExternalResetVariant=Disabled  TRSumVariant=Passthrough  SumFdbkVariant=Disabled  SumVariant=Sum_PID  TsampFilterVariant=InternalTs  TsampNgainVariant=Passthrough  TsampIntegralVariant=Disabled_SignalSpec  ExternalSaturationOutDataTypeStr=Inherit: Same as second input
  PID Controller3 : slpidlib/PID Controller  Controller=PID  Form=Parallel  TimeDomain=Continuous-time  UseExternalTs=off  SampleTime=-1  IntegratorMethod=Forward Euler  FilterMethod=Forward Euler  ControllerParametersSource=internal  P=4500  I=800  UseKiTs=off  D=8000  N=100  UseFilter=on  TunerSelectOption=Transfer Function Based (PID Tuner App)  InitialConditionSource=internal  InitialConditionForIntegrator=0  InitialConditionForFilter=0  DifferentiatorICPrevScaledInput=0  ExternalReset=none  TrackingMode=off  Kt=1  LimitOutput=off  SatLimitsSource=internal  UpperSaturationLimit=1  LowerSaturationLimit=-1  LinearizeAsGain=on  AntiWindupMode=none  Kb=1  LimitIntegrator=off  UpperIntegratorSaturationLimit=inf  LowerIntegratorSaturationLimit=-inf  POutMin=[]  POutMax=[]  IOutMin=[]  IOutMax=[]  DOutMin=[]  DOutMax=[]  NOutMin=[]  NOutMax=[]  SumOutMin=[]  SumOutMax=[]  SaturationOutMin=[]  SaturationOutMax=[]  PParamMin=[]  PParamMax=[]  IParamMin=[]  IParamMax=[]  DParamMin=[]  DParamMax=[]  NParamMin=[]  NParamMax=[]  KbParamMin=[]  KbParamMax=[]  KtParamMin=[]  KtParamMax=[]  KbOutMin=[]  KbOutMax=[]  KtOutMin=[]  KtOutMax=[]  IntegratorOutMin=[]  IntegratorOutMax=[]  FilterOutMin=[]  FilterOutMax=[]  SumI1OutMin=[]  SumI1OutMax=[]  SumI2OutMin=[]  SumI2OutMax=[]  SumI3OutMin=[]  SumI3OutMax=[]  SumI4OutMin=[]  SumI4OutMax=[]  SumDOutMin=[]  SumDOutMax=[]  DifferentiatorOutMin=[]  DifferentiatorOutMax=[]  FilterDiffOutCoefMin=[]  FilterDiffOutCoefMax=[]  ReciprocalOutMin=[]  ReciprocalOutMax=[]  SumDenOutMin=[]  SumDenOutMax=[]  SumNumOutMin=[]  SumNumOutMax=[]  DivideOutMin=[]  DivideOutMax=[]  UdiffTsProdOutMin=[]  UdiffTsProdOutMax=[]  NTsProdOutMin=[]  NTsProdOutMax=[]  UintegralTsProdOutMin=[]  UintegralTsProdOutMax=[]  UngainTsProdOutMin=[]  UngainTsProdOutMax=[]  ClampingZeroOutDataTypeStr=Inherit: Inherit via back propagation  ClampingZeroOutMin=[]  ClampingZeroOutMax=[]  FilterDenConstantOutDataTypeStr=Inherit: Inherit via back propagation  FilterDenConstantOutMin=[]  FilterDenConstantOutMax=[]  PCopyOutDataTypeStr=Inherit: Inherit via back propagation  PCopyOutMin=[]  PCopyOutMax=[]  NCopyOutDataTypeStr=Inherit: Inherit via back propagation  NCopyOutMin=[]  NCopyOutMax=[]  IntegratorContinuousStateAttributes=''  IntegratorStateMustResolveToSignalObject=off  IntegratorRTWStateStorageClass=Auto  FilterContinuousStateAttributes=''  FilterStateMustResolveToSignalObject=off  FilterRTWStateStorageClass=Auto  ParallelPVariant=InternalParameters  IdealPVariant=Disabled  IVariant=InternalParameters  DVariant=InternalParameters  IntegratorVariant=Continuous  SatVariant=Disabled  AWVariant=Passthrough  PCopyVariant=Disabled  TRVariant=Disabled  FdbkBlocksVariant=Forward  IdealPFdbkVariant=Disabled  SatFdbkVariant=Disabled  DerivativeFilterVariant=ContFilter  NVariant=InternalParameters  NCopyVariant=Disabled  FilterICVariant=InternalICsFilter  IntegratorICVariant=InternalICs  ExternalResetVariant=Disabled  TRSumVariant=Passthrough  SumFdbkVariant=Disabled  SumVariant=Sum_PID  TsampFilterVariant=InternalTs  TsampNgainVariant=Passthrough  TsampIntegralVariant=Disabled_SignalSpec  ExternalSaturationOutDataTypeStr=Inherit: Same as second input
  Product : Product
  Saturation 6V1 : Saturate  UpperLimit=5  LowerLimit=-5
  Saturation 6V2 : Saturate  UpperLimit=5  LowerLimit=-5
  Saturation 6V3 : Saturate  UpperLimit=5  LowerLimit=-5
  Scope : Scope
  Scope1 : Scope
  Scope2 : Scope
  Step : Step  Time=0  After=-1  SampleTime=0
  magTorqueMatrix : Outport
  momentoDipolar : Outport  Port=2
  wires:
  Corrección Y/1(H_error) -> PID Controller1/1
  Corrección X/1(H_error) -> PID Controller3/1
  Step/1 -> Product/2
  Campo Geomagnético1/1 -> Product/1
  Cross Product2/1 -> Add/3  "MgtZ"
  Mgt_ejeZ/1 -> Cross Product2/1
  Momento Dipolar Z/1 -> Mgt_ejeZ/1
  Saturation 6V3/1 -> Momento Dipolar Z/1  "PWR_mgt Y"
  PID Controller2/1 -> Manual Switch2/1
  Manual Switch2/1 -> Saturation 6V3/1
  MATLAB Function/2(momentoDipolar) -> Contribucion de cada Mgt2/2
  Add1/1 -> momentoDipolar/1, Contribucion de cada Mgt2/1
  MATLAB Function/1(magTorqueMatrix) -> Contribucion de cada Mgt1/2
  Add/1 -> magTorqueMatrix/1, Scope/1, Contribucion de cada Mgt1/1
  Cross Product1/1 -> Add/2, Contribucion de cada Mgt/2  "MgtY"
  Mgt_ejeY/1 -> Cross Product1/1
  Momento Dipolar Y/1 -> Mgt_ejeY/1, Add1/2
  Saturation 6V2/1 -> Momento Dipolar Y/1, MATLAB Function/3(voltageY), Scope2/1  "PWR_mgt Y"
  Cross Product/1 -> Contribucion de cada Mgt/1, Add/1  "MgtX"
  Mgt_ejeX/1 -> Cross Product/1
  Momento Dipolar X/1 -> Mgt_ejeX/1, Add1/1
  Manual Switch1/1 -> Saturation 6V1/1
  Constant1/1 -> Manual Switch1/1
  Constant/1 -> Manual Switch/2, MATLAB Function/4(voltageZ), Manual Switch2/2
  PID Controller1/1 -> Manual Switch/1
  Manual Switch/1 -> Saturation 6V2/1
  Product/1 -> Cross Product/2, Cross Product1/2, Cross Product2/2, MATLAB Function/1(B), Corrección X/2(B), Corrección Y/2(B)
  Hz_error/1 -> Corrección X/1("H_error "), Corrección Y/1("H_error "), PID Controller2/1
  Saturation 6V1/1 -> Momento Dipolar X/1, MATLAB Function/2(voltageX), Scope1/1  "PWR_mgt X"
  PID Controller3/1 -> Manual Switch1/2

== system LQR_bloques_SS_gamma/Subsystem4 ==
  euler angles : Inport
  Constant : Constant  Value=2019
  CubeSat Vehicle : aerolibcubesatveh/CubeSat Vehicle (Nadir Pointing)  sim_t0=juliandate(2019, 1, 4, 12, 0, 0)  method=Keplerian Orbital Elements  epoch=juliandate(2020, 1, 1, 12, 0, 0)  a=6786233.13  ecc=0.0010537  incl=51.7519  omega=95.2562  argp=93.4872  nu=302.9234  truelon=0  arglat=0  lonper=0  r_eci=[0 0 0]  v_eci=[0 0 0]  r_ecef=[0 0 0]  v_ecef=[0 0 0]  lla=[0 0 0]  v_ned=[0 0 0]  euler=[0 0 0]  pqr=[0 0 -0.05168]  pointingMode=Earth (Nadir) Pointing  firstAlignExt=Dialog  firstAlign=[0 0 1]  secondAlignExt=Dialog  secondAlign=[0 1 0]  constraintCoord=ECI Axes  firstRefExt=Dialog  firstRef=[1 0 0]  secondRefExt=Dialog  secondRef=[0 0 1]  missionRTSource=Dialog  missionRT=6*60*60  missionGS=[42, -71]  missionTOICheck=on  missionTOI=[]  missionEta=55
      settings: AttributesFormatString=%<pointingMode>
  Demux4 : Demux  Outputs=2
  ECEF Position to LLA : ECEF2LLA
  Environment Models : Subsystem
      mask Display:
      | port_label('input', 1, 'X_{ECEF}','texmode','on')
      | port_label('input', 2, 'V_{ECEF}','texmode','on')
      | port_label('output', 1, 'A_{ECEF}','texmode','on')
  MATLAB Function : MATLAB Function  TreatAsAtomicUnit=on
  Scope8 : Scope
  World Magnetic Model : aerolibgravity2/World Magnetic Model  model=WMM2015 V2 (2015-2020)  customFile='WMM2020.COF'  units=Metric (MKS)  time_in=on  month=January  day=1  year=2020  action=Error  h_out=on  dec_out=on  inc_out=on  ti_out=on
  nT to T : Gain  Gain=1e-9
  B : Outport
  wires:
  ECEF Position to LLA/2 -> World Magnetic Model/1
  Environment Models/1(a_ff) -> CubeSat Vehicle/1
  Constant/1 -> World Magnetic Model/4
  nT to T/1 -> MATLAB Function/1(NEDMagnetic), Scope8/1
  World Magnetic Model/1 -> nT to T/1
  CubeSat Vehicle/1 -> ECEF Position to LLA/1, Environment Models/1(x_ff)
  Demux4/2 -> World Magnetic Model/3
  euler angles/1 -> MATLAB Function/2(RPY)
  CubeSat Vehicle/2 -> Environment Models/2(v_ff)
  MATLAB Function/1(RPY_Magnetic) -> B/1
  ECEF Position to LLA/1 -> Demux4/1
  Demux4/1 -> World Magnetic Model/2

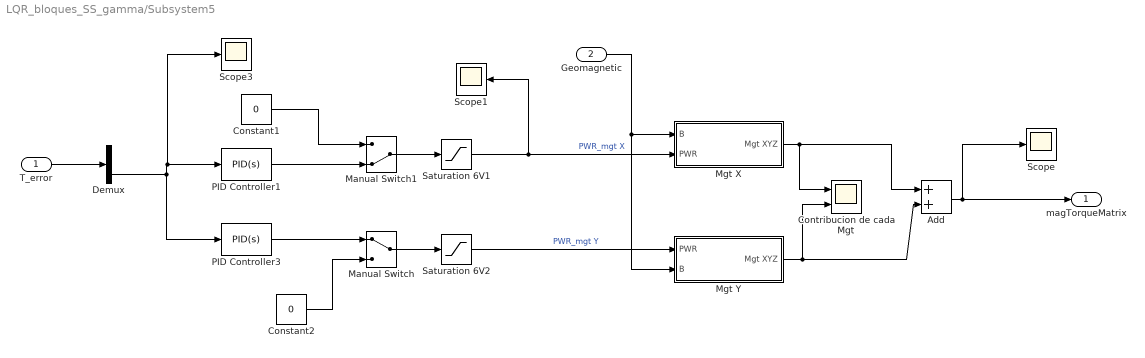
== system LQR_bloques_SS_gamma/Subsystem5 ==
  T_error : Inport
  Geomagnetic : Inport  Port=2
  Add : Sum
  Constant1 : Constant  Value=0
  Constant2 : Constant  Value=0
  Contribucion de cada Mgt : Scope  NumInputPorts=2
  Demux : Demux  Outputs=3
  Manual Switch : ManualSwitch
  Manual Switch1 : ManualSwitch  CurrentSetting=0
  Mgt X : Subsystem
  Mgt Y : Subsystem
  PID Controller1 : slpidlib/PID Controller  Controller=PID  Form=Parallel  TimeDomain=Continuous-time  UseExternalTs=off  SampleTime=-1  IntegratorMethod=Forward Euler  FilterMethod=Forward Euler  ControllerParametersSource=internal  P=500000  I=30000  UseKiTs=off  D=2500  N=100  UseFilter=on  TunerSelectOption=Transfer Function Based (PID Tuner App)  InitialConditionSource=internal  InitialConditionForIntegrator=0  InitialConditionForFilter=0  DifferentiatorICPrevScaledInput=0  ExternalReset=none  TrackingMode=off  Kt=1  LimitOutput=off  SatLimitsSource=internal  UpperSaturationLimit=1  LowerSaturationLimit=-1  LinearizeAsGain=on  AntiWindupMode=none  Kb=1  LimitIntegrator=off  UpperIntegratorSaturationLimit=inf  LowerIntegratorSaturationLimit=-inf  POutMin=[]  POutMax=[]  IOutMin=[]  IOutMax=[]  DOutMin=[]  DOutMax=[]  NOutMin=[]  NOutMax=[]  SumOutMin=[]  SumOutMax=[]  SaturationOutMin=[]  SaturationOutMax=[]  PParamMin=[]  PParamMax=[]  IParamMin=[]  IParamMax=[]  DParamMin=[]  DParamMax=[]  NParamMin=[]  NParamMax=[]  KbParamMin=[]  KbParamMax=[]  KtParamMin=[]  KtParamMax=[]  KbOutMin=[]  KbOutMax=[]  KtOutMin=[]  KtOutMax=[]  IntegratorOutMin=[]  IntegratorOutMax=[]  FilterOutMin=[]  FilterOutMax=[]  SumI1OutMin=[]  SumI1OutMax=[]  SumI2OutMin=[]  SumI2OutMax=[]  SumI3OutMin=[]  SumI3OutMax=[]  SumI4OutMin=[]  SumI4OutMax=[]  SumDOutMin=[]  SumDOutMax=[]  DifferentiatorOutMin=[]  DifferentiatorOutMax=[]  FilterDiffOutCoefMin=[]  FilterDiffOutCoefMax=[]  ReciprocalOutMin=[]  ReciprocalOutMax=[]  SumDenOutMin=[]  SumDenOutMax=[]  SumNumOutMin=[]  SumNumOutMax=[]  DivideOutMin=[]  DivideOutMax=[]  UdiffTsProdOutMin=[]  UdiffTsProdOutMax=[]  NTsProdOutMin=[]  NTsProdOutMax=[]  UintegralTsProdOutMin=[]  UintegralTsProdOutMax=[]  UngainTsProdOutMin=[]  UngainTsProdOutMax=[]  ClampingZeroOutDataTypeStr=Inherit: Inherit via back propagation  ClampingZeroOutMin=[]  ClampingZeroOutMax=[]  FilterDenConstantOutDataTypeStr=Inherit: Inherit via back propagation  FilterDenConstantOutMin=[]  FilterDenConstantOutMax=[]  PCopyOutDataTypeStr=Inherit: Inherit via back propagation  PCopyOutMin=[]  PCopyOutMax=[]  NCopyOutDataTypeStr=Inherit: Inherit via back propagation  NCopyOutMin=[]  NCopyOutMax=[]  IntegratorContinuousStateAttributes=''  IntegratorStateMustResolveToSignalObject=off  IntegratorRTWStateStorageClass=Auto  FilterContinuousStateAttributes=''  FilterStateMustResolveToSignalObject=off  FilterRTWStateStorageClass=Auto  ParallelPVariant=InternalParameters  IdealPVariant=Disabled  IVariant=InternalParameters  DVariant=InternalParameters  IntegratorVariant=Continuous  SatVariant=Disabled  AWVariant=Passthrough  PCopyVariant=Disabled  TRVariant=Disabled  FdbkBlocksVariant=Forward  IdealPFdbkVariant=Disabled  SatFdbkVariant=Disabled  DerivativeFilterVariant=ContFilter  NVariant=InternalParameters  NCopyVariant=Disabled  FilterICVariant=InternalICsFilter  IntegratorICVariant=InternalICs  ExternalResetVariant=Disabled  TRSumVariant=Passthrough  SumFdbkVariant=Disabled  SumVariant=Sum_PID  TsampFilterVariant=InternalTs  TsampNgainVariant=Passthrough  TsampIntegralVariant=Disabled_SignalSpec  ExternalSaturationOutDataTypeStr=Inherit: Same as second input
  PID Controller3 : slpidlib/PID Controller  Controller=PID  Form=Parallel  TimeDomain=Continuous-time  UseExternalTs=off  SampleTime=-1  IntegratorMethod=Forward Euler  FilterMethod=Forward Euler  ControllerParametersSource=internal  P=500000  I=30000  UseKiTs=off  D=2500  N=100  UseFilter=on  TunerSelectOption=Transfer Function Based (PID Tuner App)  InitialConditionSource=internal  InitialConditionForIntegrator=0  InitialConditionForFilter=0  DifferentiatorICPrevScaledInput=0  ExternalReset=none  TrackingMode=off  Kt=1  LimitOutput=off  SatLimitsSource=internal  UpperSaturationLimit=1  LowerSaturationLimit=-1  LinearizeAsGain=on  AntiWindupMode=none  Kb=1  LimitIntegrator=off  UpperIntegratorSaturationLimit=inf  LowerIntegratorSaturationLimit=-inf  POutMin=[]  POutMax=[]  IOutMin=[]  IOutMax=[]  DOutMin=[]  DOutMax=[]  NOutMin=[]  NOutMax=[]  SumOutMin=[]  SumOutMax=[]  SaturationOutMin=[]  SaturationOutMax=[]  PParamMin=[]  PParamMax=[]  IParamMin=[]  IParamMax=[]  DParamMin=[]  DParamMax=[]  NParamMin=[]  NParamMax=[]  KbParamMin=[]  KbParamMax=[]  KtParamMin=[]  KtParamMax=[]  KbOutMin=[]  KbOutMax=[]  KtOutMin=[]  KtOutMax=[]  IntegratorOutMin=[]  IntegratorOutMax=[]  FilterOutMin=[]  FilterOutMax=[]  SumI1OutMin=[]  SumI1OutMax=[]  SumI2OutMin=[]  SumI2OutMax=[]  SumI3OutMin=[]  SumI3OutMax=[]  SumI4OutMin=[]  SumI4OutMax=[]  SumDOutMin=[]  SumDOutMax=[]  DifferentiatorOutMin=[]  DifferentiatorOutMax=[]  FilterDiffOutCoefMin=[]  FilterDiffOutCoefMax=[]  ReciprocalOutMin=[]  ReciprocalOutMax=[]  SumDenOutMin=[]  SumDenOutMax=[]  SumNumOutMin=[]  SumNumOutMax=[]  DivideOutMin=[]  DivideOutMax=[]  UdiffTsProdOutMin=[]  UdiffTsProdOutMax=[]  NTsProdOutMin=[]  NTsProdOutMax=[]  UintegralTsProdOutMin=[]  UintegralTsProdOutMax=[]  UngainTsProdOutMin=[]  UngainTsProdOutMax=[]  ClampingZeroOutDataTypeStr=Inherit: Inherit via back propagation  ClampingZeroOutMin=[]  ClampingZeroOutMax=[]  FilterDenConstantOutDataTypeStr=Inherit: Inherit via back propagation  FilterDenConstantOutMin=[]  FilterDenConstantOutMax=[]  PCopyOutDataTypeStr=Inherit: Inherit via back propagation  PCopyOutMin=[]  PCopyOutMax=[]  NCopyOutDataTypeStr=Inherit: Inherit via back propagation  NCopyOutMin=[]  NCopyOutMax=[]  IntegratorContinuousStateAttributes=''  IntegratorStateMustResolveToSignalObject=off  IntegratorRTWStateStorageClass=Auto  FilterContinuousStateAttributes=''  FilterStateMustResolveToSignalObject=off  FilterRTWStateStorageClass=Auto  ParallelPVariant=InternalParameters  IdealPVariant=Disabled  IVariant=InternalParameters  DVariant=InternalParameters  IntegratorVariant=Continuous  SatVariant=Disabled  AWVariant=Passthrough  PCopyVariant=Disabled  TRVariant=Disabled  FdbkBlocksVariant=Forward  IdealPFdbkVariant=Disabled  SatFdbkVariant=Disabled  DerivativeFilterVariant=ContFilter  NVariant=InternalParameters  NCopyVariant=Disabled  FilterICVariant=InternalICsFilter  IntegratorICVariant=InternalICs  ExternalResetVariant=Disabled  TRSumVariant=Passthrough  SumFdbkVariant=Disabled  SumVariant=Sum_PID  TsampFilterVariant=InternalTs  TsampNgainVariant=Passthrough  TsampIntegralVariant=Disabled_SignalSpec  ExternalSaturationOutDataTypeStr=Inherit: Same as second input
  Saturation 6V1 : Saturate  UpperLimit=3  LowerLimit=-3
  Saturation 6V2 : Saturate  UpperLimit=5  LowerLimit=-5
  Scope : Scope
  Scope1 : Scope
  Scope3 : Scope
  magTorqueMatrix : Outport
  wires:
  PID Controller1/1 -> Manual Switch1/2
  Saturation 6V1/1 -> Mgt X/2(PWR), Scope1/1  "PWR_mgt X"
  Geomagnetic/1 -> Mgt Y/2(B), Mgt X/1(B)
  Manual Switch/1 -> Saturation 6V2/1
  PID Controller3/1 -> Manual Switch/1
  Constant1/1 -> Manual Switch1/1
  Manual Switch1/1 -> Saturation 6V1/1
  Saturation 6V2/1 -> Mgt Y/1(PWR)  "PWR_mgt Y"
  Add/1 -> Scope/1, magTorqueMatrix/1
  T_error/1 -> Demux/1
  Mgt X/1(Mgt XYZ) -> Contribucion de cada Mgt/1, Add/1
  Mgt Y/1(Mgt XYZ) -> Add/2, Contribucion de cada Mgt/2
  Constant2/1 -> Manual Switch/2
  Demux/3 -> PID Controller3/1, PID Controller1/1, Scope3/1
